simulink model "continuous_battery"  (R2020a)
settings: Solver=ode4  StartTime=0.0  StopTime=20000  FixedStep=.1  RelTol=1e-3
undefined symbols (not defined in the file): uav
settings Model: Creator=darrahts  LastModifiedBy=darrahts
settings OptimizationCC: DefaultUnderspecifiedDataType=single
settings DebuggingCC: SignalInfNanChecking=warning  Int32ToFloatConvMsg=none  ParameterDowncastMsg=warning  FixptConstPrecisionLossMsg=warning

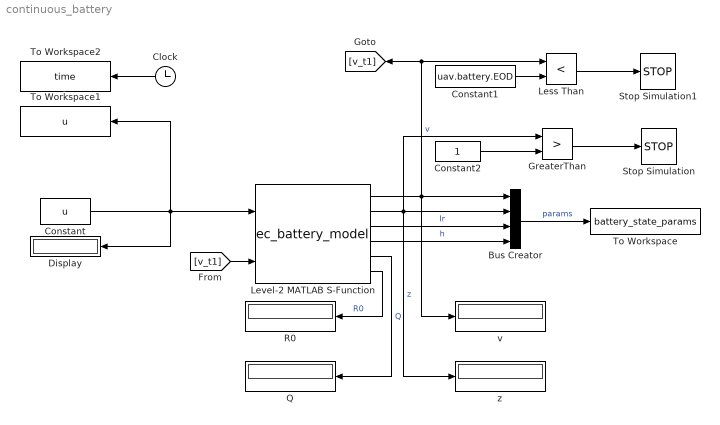
== system continuous_battery ==
  Bus Creator : BusCreator  Inputs=4
  Clock : Clock
  Constant : Constant  Value=u
  Constant1 : Constant  Value=uav.battery.EOD
  Constant2 : Constant
  Display : Display
  GreaterThan : RelationalOperator  Operator=>  OutDataTypeStr=boolean  RndMeth=Simplest
  Less Than : RelationalOperator  Operator=<  OutDataTypeStr=boolean  RndMeth=Simplest
  Level-2 MATLAB S-Function : M-S-Function  FunctionName=ec_battery_model  Parameters=uav.battery
      mask Display:
      | port_label('output', 1, 'v');
      | port_label('output', 2, 'z');
      | port_label('output', 3, 'Ir');
      | port_label('output', 4, 'h');
      | port_label('output', 5, 'Q');
      | port_label('output', 6, 'R0');
      | 
      | port_label('input', 1, 'u');
      | port_label('input', 2, 'v_(t-1)');
  Q : Display
  R0 : Display
  Stop Simulation : Stop
  Stop Simulation1 : Stop
  To Workspace : ToWorkspace  VariableName=battery_state_params  SaveFormat=Timeseries  SampleTime=-1
  To Workspace1 : ToWorkspace  VariableName=u  SaveFormat=Timeseries  SampleTime=-1
  To Workspace2 : ToWorkspace  VariableName=time  SaveFormat=Timeseries  SampleTime=-1
  v : Display
  z : Display
  wires:
  Level-2 MATLAB S-Function/1 -> v/1, Bus Creator/1, [v_t1], Less Than/1  "v"
  Constant/1 -> Display/1, Level-2 MATLAB S-Function/1, To Workspace1/1
  Level-2 MATLAB S-Function/2 -> z/1, Bus Creator/2, GreaterThan/1  "z"
  Bus Creator/1 -> To Workspace/1  "params"
  Level-2 MATLAB S-Function/3 -> Bus Creator/3  "Ir"
  Level-2 MATLAB S-Function/4 -> Bus Creator/4  "h"
  Level-2 MATLAB S-Function/5 -> Q/1  "Q"
  Clock/1 -> To Workspace2/1
  Constant1/1 -> Less Than/2
  Constant2/1 -> GreaterThan/2
  GreaterThan/1 -> Stop Simulation/1
  Less Than/1 -> Stop Simulation1/1
  Level-2 MATLAB S-Function/6 -> R0/1  "R0"
  [v_t1] -> Level-2 MATLAB S-Function/2
